simulink model "RPLANT"  (R2017a)
settings: Solver=VariableStepAuto  StartTime=0.0  StopTime=10.0  RelTol=1e-3
values from neighbouring files (symbols this model uses):
  g = 9.80665    [automatas_matlab.m]
undefined symbols (not defined in the file or in its folder): bh, bt, bw, Kw, Mh, Mt, rt, Rw, yt, yt0
settings Model: Creator=elust  LastModifiedBy=elust

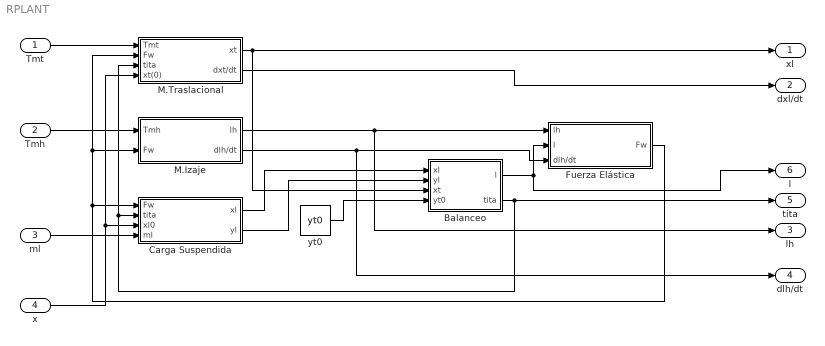
== system RPLANT ==
  Tmt : Inport
  Tmh : Inport  Port=2
  ml : Inport  Port=3
  x : Inport  Port=4
  Balanceo : MATLAB Function  TreatAsAtomicUnit=on
  Carga Suspendida : Subsystem
  Fuerza Elástica : Subsystem
  M.Izaje : Subsystem
  M.Traslacional : Subsystem
  yt0 : Constant  Value=yt0
  xl : Outport
  dxl/dt : Outport  Port=2
  lh : Outport  Port=3
  dlh/dt : Outport  Port=4
  tita : Outport  Port=5
  l : Outport  Port=6
  wires:
  Tmh/1 -> M.Izaje/1(Tmh)
  Tmt/1 -> M.Traslacional/1("Tmt ")
  ml/1 -> Carga Suspendida/4(ml)
  Balanceo/1(l) -> l/1, Fuerza Elástica/2(l)
  M.Izaje/1(lh) -> Fuerza Elástica/1(lh), lh/1
  M.Izaje/2(dlh/dt) -> Fuerza Elástica/3(dlh/dt), dlh/dt/1
  Carga Suspendida/1(xl) -> Balanceo/1(xl)
  Carga Suspendida/2(yl) -> Balanceo/2(yl)
  Fuerza Elástica/1(Fw) -> M.Traslacional/2(Fw), M.Izaje/2(Fw), Carga Suspendida/1(Fw)
  M.Traslacional/1(xt) -> xl/1, Balanceo/3(xt)
  M.Traslacional/2(dxt/dt) -> dxl/dt/1
  yt0/1 -> Balanceo/4(yt0)
  Balanceo/2(tita) -> tita/1, M.Traslacional/3(tita), Carga Suspendida/2(tita)
  x/1 -> Carga Suspendida/3(xl0), M.Traslacional/4(xt(0))

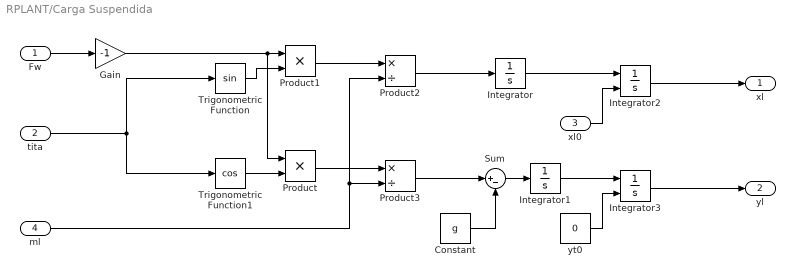
== system RPLANT/Carga Suspendida ==
  Fw : Inport
  tita : Inport  Port=2
  xl0 : Inport  Port=3
  ml : Inport  Port=4
  Constant : Constant  Value=g
  Gain : Gain  Gain=-1
  Integrator : Integrator
  Integrator1 : Integrator
  Integrator2 : Integrator  InitialConditionSource=external
  Integrator3 : Integrator  InitialConditionSource=external
  Product : Product
  Product1 : Product
  Product2 : Product  Inputs=*/
  Product3 : Product  Inputs=*/
  Sum : Sum  Inputs=|+-
  Trigonometric Function : Trigonometry
  Trigonometric Function1 : Trigonometry  Operator=cos
  yt0 : Constant  Value=0
  xl : Outport
  yl : Outport  Port=2
  wires:
  tita/1 -> Trigonometric Function/1, Trigonometric Function1/1
  Constant/1 -> Sum/2
  Trigonometric Function1/1 -> Product/2
  Fw/1 -> Gain/1
  Trigonometric Function/1 -> Product1/2
  Sum/1 -> Integrator1/1
  Integrator/1 -> Integrator2/1
  Integrator1/1 -> Integrator3/1
  yt0/1 -> Integrator3/2
  xl0/1 -> Integrator2/2
  Integrator2/1 -> xl/1
  Integrator3/1 -> yl/1
  Product/1 -> Product3/1
  Product1/1 -> Product2/1
  ml/1 -> Product2/2, Product3/2
  Product2/1 -> Integrator/1
  Product3/1 -> Sum/1
  Gain/1 -> Product1/1, Product/1

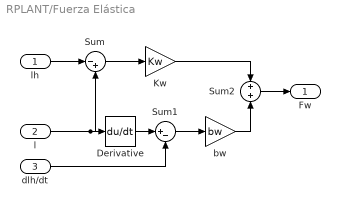
== system RPLANT/Fuerza Elástica ==
  lh : Inport
  l : Inport  Port=2
  dlh/dt : Inport  Port=3
  Derivative : Derivative
  Kw : Gain  Gain=Kw
  Sum : Sum  Inputs=|-+
  Sum1 : Sum  Inputs=|+-
  Sum2 : Sum
  bw : Gain  Gain=bw
  Fw : Outport
  wires:
  l/1 -> Sum/2, Derivative/1
  lh/1 -> Sum/1
  Sum/1 -> Kw/1
  Derivative/1 -> Sum1/1
  dlh/dt/1 -> Sum1/2
  Sum1/1 -> bw/1
  Sum2/1 -> Fw/1
  Kw/1 -> Sum2/1
  bw/1 -> Sum2/2

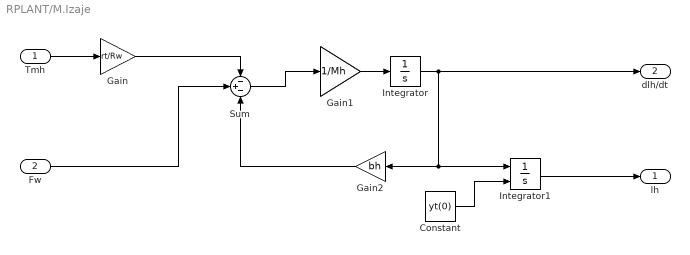
== system RPLANT/M.Izaje ==
  Tmh : Inport
  Fw : Inport  Port=2
  Constant : Constant  Value=yt(0)
  Gain : Gain  Gain=rt/Rw
  Gain1 : Gain  Gain=1/Mh
  Gain2 : Gain  Gain=bh
  Integrator : Integrator
  Integrator1 : Integrator  InitialConditionSource=external
  Sum : Sum  Inputs=-+-
  lh : Outport
  dlh/dt : Outport  Port=2
  wires:
  Tmh/1 -> Gain/1
  Gain/1 -> Sum/1
  Sum/1 -> Gain1/1
  Gain1/1 -> Integrator/1
  Integrator/1 -> dlh/dt/1, Integrator1/1, Gain2/1
  Gain2/1 -> Sum/3
  Fw/1 -> Sum/2
  Constant/1 -> Integrator1/2
  Integrator1/1 -> lh/1

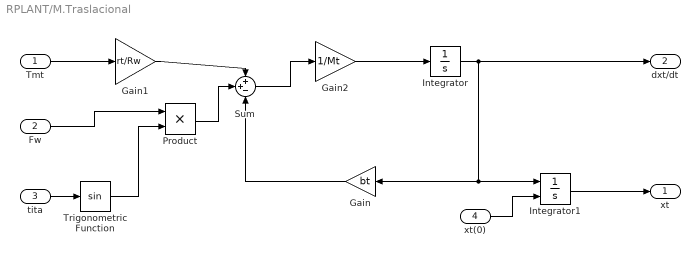
== system RPLANT/M.Traslacional ==
  "Tmt " : Inport
  Fw : Inport  Port=2
  tita : Inport  Port=3
  xt(0) : Inport  Port=4
  Gain : Gain  Gain=bt
  Gain1 : Gain  Gain=rt/Rw
  Gain2 : Gain  Gain=1/Mt
  Integrator : Integrator
  Integrator1 : Integrator  InitialConditionSource=external
  Product : Product
  Sum : Sum  Inputs=++-
  Trigonometric Function : Trigonometry
  xt : Outport
  dxt/dt : Outport  Port=2
  wires:
  Gain2/1 -> Integrator/1
  Trigonometric Function/1 -> Product/2
  tita/1 -> Trigonometric Function/1
  Integrator/1 -> dxt/dt/1, Integrator1/1, Gain/1
  Gain/1 -> Sum/3
  Fw/1 -> Product/1
  Product/1 -> Sum/2
  Sum/1 -> Gain2/1
  Gain1/1 -> Sum/1
  xt(0)/1 -> Integrator1/2
  "Tmt "/1 -> Gain1/1
  Integrator1/1 -> xt/1

== matlab function RPLANT/Balanceo ==
  data: xl input; l output; yl input; xt input; yt0 input; tita output
function [l,tita] = fcn(xl,yl,xt,yt0)

deltax = (x1-x0)
deltay = (y1-yt0)


l = sqrt((deltax^2)+(deltay^2));

tita = atan2(deltax/deltay);

end;
